simulink model "Exemplu5_a_si_b"  (R2021b)
settings: Solver=VariableStepAuto  StartTime=0.0  StopTime=20  RelTol=1e-3
settings Model: Creator=alexandra.szedlak-st  LastModifiedBy=alexandra.szedlak-st

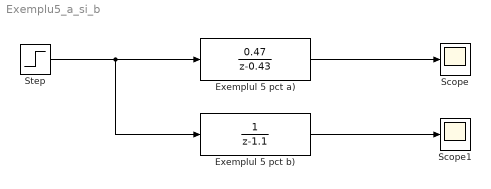
== system Exemplu5_a_si_b ==
  Exemplul 5 pct a) : DiscreteTransferFcn  Numerator=[0.47]  Denominator=[1 -0.43]  SampleTime=0.05
  Exemplul 5 pct b) : DiscreteTransferFcn  Denominator=[1 -1.1]  SampleTime=0.05
  Scope : Scope
  Scope1 : Scope
  Step : Step  Time=0  After=5  SampleTime=0
  wires:
  Exemplul 5 pct a)/1 -> Scope/1
  Exemplul 5 pct b)/1 -> Scope1/1
  Step/1 -> Exemplul 5 pct a)/1, Exemplul 5 pct b)/1
